simulink subsystem "Average_SEPIC"  (R2021b)
settings: Solver=VariableStepAuto  StartTime=0.0  StopTime=0.5  RelTol=1e-3
undefined symbols (not defined in the file): D1_Rs, D1_Vf, PR1_Res, R9_Res
libraries: fl_lib x23, ee_lib x7, nesl_utility x5, simulink x1
settings Model: DefaultTestHarness=DCDC_SEPIC_Pulse0_61_LED0  Creator=vlenzi  LastModifiedBy=vlenzi
settings SolverCC: AlgebraicLoopSolver=TrustRegion
settings DebuggingCC: SFMachineParentedDataDiag=warning

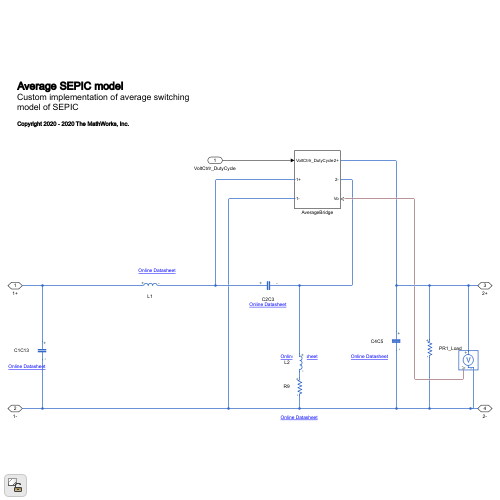
[thumbnail: Simulink's stored preview of the top-level diagram]
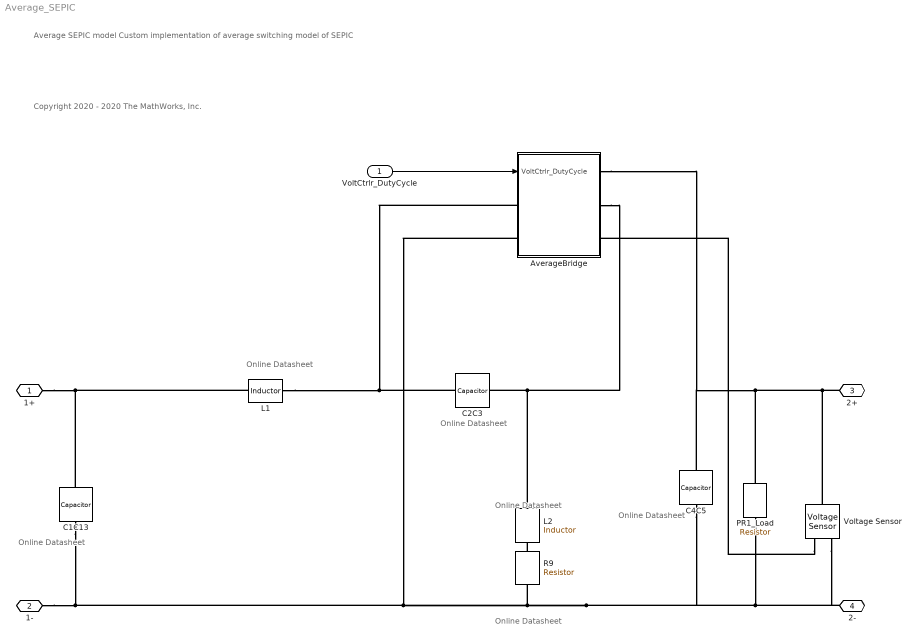
== system Average_SEPIC ==
  note: Online Datasheet
  note: Online Datasheet
  note: Online Datasheet
  note: Online Datasheet
  note: Online Datasheet
  note: Online Datasheet
  note: Average SEPIC model
      | Custom implementation of average switching model of SEPIC
  note: Copyright 2020 - 2020 The MathWorks, Inc.
  VoltCtrlr_DutyCycle : Inport  Unit=1  PortDimensions=1
  AverageBridge : Subsystem
  C1C13 : ee_lib/Passive/Capacitor  cap_option=0  c=C1C13_Cap uF  Cvec=[1e-05, 1e-06] F  Vvec=[0, 10] V  CV_table_symmetry=1  f_vec=[1, 10] kHz  DFext_vec=[.8, 1.2]  C_tol=C1C13_Tol  enable_C_tol=0  tol_distribution=1  nSigma=4  r=1e-6 Ohm  g=0 1/Ohm  averaging_period=0 s  enable_operating_limits=0  operating_limit_action=2  max_working_voltage_range=[-25, 25] V  power_rating=1 W  enable_faults=0  fault_action=1  Cscale_faulted=100  R_faulted=1e-3 Ohm  G_faulted=0 1/Ohm  tau_fault=1e-3 s  enable_temporal_fault=0  t_fault=1 s  enable_behavioral_fault=0  max_permissible_voltage_range=[-100, 100] V  t_fail_on_voltage=1 s  i_specify=off  i_priority=None  i=0 A  i_nominal_specify=off  i_nominal_unit=A  i_nominal_value=1  v_specify=off  v_priority=None  v=0 V  v_nominal_specify=off  v_nominal_unit=V  v_nominal_value=1  vc_specify=off  vc_priority=High  vc=0 V  vc_nominal_specify=off  vc_nominal_unit=V  vc_nominal_value=1
  C2C3 : ee_lib/Passive/Capacitor  cap_option=0  c=C2C3_Cap uF  Cvec=[1e-05, 1e-06] F  Vvec=[0, 10] V  CV_table_symmetry=1  f_vec=[1, 10] kHz  DFext_vec=[.8, 1.2]  C_tol=C2C3_Tol  enable_C_tol=0  tol_distribution=1  nSigma=4  r=1e-6 Ohm  g=0 1/Ohm  averaging_period=0 s  enable_operating_limits=0  operating_limit_action=2  max_working_voltage_range=[-25, 25] V  power_rating=1 W  enable_faults=0  fault_action=1  Cscale_faulted=100  R_faulted=1e-3 Ohm  G_faulted=0 1/Ohm  tau_fault=1e-3 s  enable_temporal_fault=0  t_fault=1 s  enable_behavioral_fault=0  max_permissible_voltage_range=[-100, 100] V  t_fail_on_voltage=1 s  i_specify=off  i_priority=None  i=0 A  i_nominal_specify=off  i_nominal_unit=A  i_nominal_value=1  v_specify=off  v_priority=High  v=psu_V V  v_nominal_specify=off  v_nominal_unit=V  v_nominal_value=1  vc_specify=off  vc_priority=High  vc=0 V  vc_nominal_specify=off  vc_nominal_unit=V  vc_nominal_value=1
  C4C5 : ee_lib/Passive/Capacitor  cap_option=0  c=C4C5_Cap uF  Cvec=[1e-05, 1e-06] F  Vvec=[0, 10] V  CV_table_symmetry=1  f_vec=[1, 10] kHz  DFext_vec=[.8, 1.2]  C_tol=C4C5_Tol  enable_C_tol=0  tol_distribution=1  nSigma=4  r=1e-6 Ohm  g=0 1/Ohm  averaging_period=0 s  enable_operating_limits=0  operating_limit_action=2  max_working_voltage_range=[-25, 25] V  power_rating=1 W  enable_faults=0  fault_action=1  Cscale_faulted=100  R_faulted=1e-3 Ohm  G_faulted=0 1/Ohm  tau_fault=1e-3 s  enable_temporal_fault=0  t_fault=1 s  enable_behavioral_fault=0  max_permissible_voltage_range=[-100, 100] V  t_fail_on_voltage=1 s  i_specify=off  i_priority=None  i=0 A  i_nominal_specify=off  i_nominal_unit=A  i_nominal_value=1  v_specify=off  v_priority=None  v=0 V  v_nominal_specify=off  v_nominal_unit=V  v_nominal_value=1  vc_specify=off  vc_priority=High  vc=0 V  vc_nominal_specify=off  vc_nominal_unit=V  vc_nominal_value=1
  L1 : ee_lib/Passive/Inductor  l=L1_Ind uH  L_tol=L1_Tol  enable_L_tol=0  tol_distribution=1  nSigma=4  r=L1_Res Ohm  g=0 1/Ohm  enable_operating_limits=0  operating_limit_action=2  max_working_current=1 A  power_rating=1 W  enable_faults=0  fault_action=1  lambdaPercent=50  k_faulted=0.9999  turnsShort=0  openCct=0  groundShort=0  groundShortG=0 1/Ohm  tau_fault=1e-3 s  enable_temporal_fault=0  t_fault=1 s  enable_behavioral_fault=0  max_permissible_voltage=100 V  n_fail_on_voltage=1  max_permissible_current=1 A  t_fail_on_current=1 s  i_L_specify=off  i_L_priority=High  i_L=0 A  i_L_nominal_specify=off  i_L_nominal_unit=A  i_L_nominal_value=1
  L2 : ee_lib/Passive/Inductor  l=L2_Ind uH  L_tol=L2_Tol  enable_L_tol=0  tol_distribution=1  nSigma=4  r=L2_Res Ohm  g=0 1/Ohm  enable_operating_limits=0  operating_limit_action=2  max_working_current=1 A  power_rating=1 W  enable_faults=0  fault_action=1  lambdaPercent=50  k_faulted=0.9999  turnsShort=0  openCct=0  groundShort=0  groundShortG=0 1/Ohm  tau_fault=1e-3 s  enable_temporal_fault=0  t_fault=1 s  enable_behavioral_fault=0  max_permissible_voltage=100 V  n_fail_on_voltage=1  max_permissible_current=1 A  t_fail_on_current=1 s  i_L_specify=off  i_L_priority=High  i_L=0 A  i_L_nominal_specify=off  i_L_nominal_unit=A  i_L_nominal_value=1
  PR1_Load : ee_lib/Passive/Resistor  R=PR1_Res Ohm  R_tol=PR1_Tol  enable_R_tol=0  tol_distribution=1  nSigma=4  enable_operating_limits=0  operating_limit_action=2  max_working_voltage=100 V  power_rating=1 W  enable_faults=0  fault_action=1  R_faulted=inf Ohm  enable_temporal_fault=0  t_fault=1 s  enable_behavioral_fault=0  max_permissible_current=1 A  t_fail_on_current=1 s  noise_mode=0  sample_time=1e-3 s  repeatability=1  auto_seed=3118594787  user_seed=0  Tdevice=25 degC  power_derating_T1=70 degC  power_derating_T2=155 degC  operating_temperature_range_vec=[-50, 150] degC  alpha=3.93e-3 1/K  Tmeas=25 degC  thermal_mass=100 J/K  temperature_specify=off  temperature_priority=High  temperature=298.15 K  temperature_nominal_specify=off  temperature_nominal_unit=K  temperature_nominal_value=1
  R9 : ee_lib/Passive/Resistor  R=R9_Res Ohm  R_tol=R9_Tol  enable_R_tol=0  tol_distribution=1  nSigma=4  enable_operating_limits=0  operating_limit_action=2  max_working_voltage=100 V  power_rating=1 W  enable_faults=0  fault_action=1  R_faulted=inf Ohm  enable_temporal_fault=0  t_fault=1 s  enable_behavioral_fault=0  max_permissible_current=1 A  t_fail_on_current=1 s  noise_mode=0  sample_time=1e-3 s  repeatability=1  auto_seed=3362409950  user_seed=0  Tdevice=25 degC  power_derating_T1=70 degC  power_derating_T2=155 degC  operating_temperature_range_vec=[-50, 150] degC  alpha=3.93e-3 1/K  Tmeas=25 degC  thermal_mass=100 J/K  temperature_specify=off  temperature_priority=High  temperature=298.15 K  temperature_nominal_specify=off  temperature_nominal_unit=K  temperature_nominal_value=1
  Voltage Sensor : fl_lib/Electrical/Electrical Sensors/Voltage Sensor
  1+ : PMIOPort  Side=Left
  1- : PMIOPort  Port=2  Side=Left
  2+ : PMIOPort  Port=3  Side=Right
  2- : PMIOPort  Port=4  Side=Right
  wires:
  VoltCtrlr_DutyCycle/1 -> AverageBridge/1(VoltCtrlr_DutyCycle)
  connections:
  Voltage Sensor/LConn1 -- AverageBridge/RConn1 -- C4C5/LConn1 -- PR1_Load/LConn1 -- 2+/RConn1
  L1/LConn1 -- C1C13/LConn1 -- 1+/RConn1
  1-/RConn1 -- 2-/RConn1 -- Voltage Sensor/RConn2 -- PR1_Load/RConn1 -- C4C5/RConn1 -- R9/RConn1 -- AverageBridge/LConn2 -- C1C13/RConn1
  AverageBridge/LConn1 -- C2C3/LConn1 -- L1/RConn1
  L2/LConn1 -- C2C3/RConn1 -- AverageBridge/RConn2
  R9/LConn1 -- L2/RConn1
  Voltage Sensor/RConn1 -- AverageBridge/RConn3

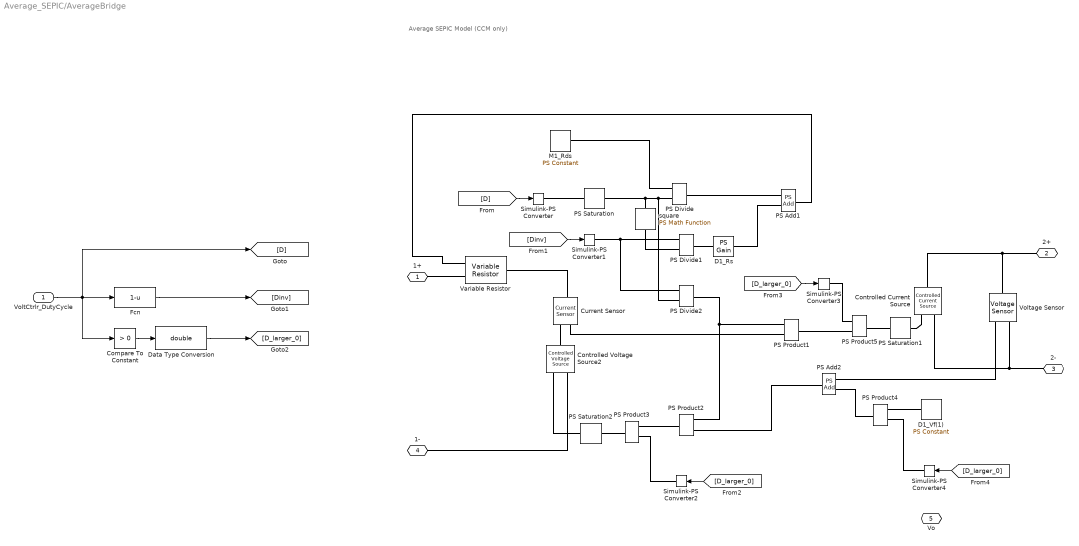
== system Average_SEPIC/AverageBridge ==
  note: Average SEPIC Model (CCM only)
  VoltCtrlr_DutyCycle : Inport  Unit=1  PortDimensions=1
  Compare To Constant : simulink/Logic and Bit Operations/Compare To Constant  relop=>  const=0  OutDataTypeStr=uint8
  Controlled Current Source : fl_lib/Electrical/Electrical Sources/Controlled Current Source
  Controlled Voltage Source2 : fl_lib/Electrical/Electrical Sources/Controlled Voltage Source
  Current Sensor : fl_lib/Electrical/Electrical Sensors/Current Sensor
  D1_Rs : fl_lib/Physical Signals/Functions/PS Gain  gain=D1_Rs Ohm
  D1_Vf(1) : fl_lib/Physical Signals/Sources/PS Constant  constant=D1_Vf(1) V
  Data Type Conversion : DataTypeConversion  OutDataTypeStr=double
  Fcn : Fcn  Expr=1-u
  M1_Rds : fl_lib/Physical Signals/Sources/PS Constant  constant=M1_Rds Ohm
  PS Add1 : fl_lib/Physical Signals/Functions/PS Add
  PS Add2 : fl_lib/Physical Signals/Functions/PS Add
  PS Divide : fl_lib/Physical Signals/Functions/PS Divide
      settings: SourceProductBaseCode=SS
  PS Divide1 : fl_lib/Physical Signals/Functions/PS Divide
      settings: SourceProductBaseCode=SS
  PS Divide2 : fl_lib/Physical Signals/Functions/PS Divide
      settings: SourceProductBaseCode=SS
  PS Product{1..5} (5 alike) : fl_lib/Physical Signals/Functions/PS Product
  PS Saturation : fl_lib/Physical Signals/Nonlinear Operators/PS Saturation  upper_limit=inf  lower_limit=1e-5
      settings: SourceProductBaseCode=SS
  PS Saturation1 : fl_lib/Physical Signals/Nonlinear Operators/PS Saturation  upper_limit=inf A  lower_limit=0 A
      settings: SourceProductBaseCode=SS
  PS Saturation2 : fl_lib/Physical Signals/Nonlinear Operators/PS Saturation  upper_limit=inf V  lower_limit=0 V
      settings: SourceProductBaseCode=SS
  Simulink-PS Converter{,1..4} (5 alike) : nesl_utility/Simulink-PS Converter  PhysicalDomain=network_engine_domain  SubClassName=ps_input  LeftPortType=input  RightPortType=output  PseudoPeriodic=off  Frequencies=[]  NoiseDistribution=none  NoiseParameters=[]  Unit=1  AffineConversion=off  FilteringAndDerivatives=provide  SimscapeFilterOrder=1  InputFilterTimeConstant=0.001  UdotUserProvided=0
      settings: SourceProductBaseCode=PW,SS
  Variable Resistor : fl_lib/Electrical/Electrical Elements/Variable Resistor  Rmin=0 Ohm  i_specify=off  i_priority=None  i=0 A  i_nominal_specify=off  i_nominal_unit=A  i_nominal_value=1  v_specify=off  v_priority=None  v=0 V  v_nominal_specify=off  v_nominal_unit=V  v_nominal_value=1
  Voltage Sensor : fl_lib/Electrical/Electrical Sensors/Voltage Sensor
  square : fl_lib/Physical Signals/Functions/PS Math Function  fcn_choice=foundation.enum.math_function.square  v=1
      settings: SourceProductBaseCode=SS
  1+ : PMIOPort  Side=Left
  2+ : PMIOPort  Port=2  Side=Right
  2- : PMIOPort  Port=3  Side=Right
  1- : PMIOPort  Port=4  Side=Left
  Vo : PMIOPort  Port=5  Side=Right
  wires:
  VoltCtrlr_DutyCycle/1 -> Compare To Constant/1, Fcn/1, [D]
  Fcn/1 -> [Dinv]
  Compare To Constant/1 -> Data Type Conversion/1
  Data Type Conversion/1 -> [D_larger_0]
  [D] -> Simulink-PS Converter/1
  [Dinv] -> Simulink-PS Converter1/1
  [D_larger_0] -> Simulink-PS Converter2/1
  [D_larger_0] -> Simulink-PS Converter3/1
  [D_larger_0] -> Simulink-PS Converter4/1
  connections:
  Current Sensor/RConn1 -- PS Product1/LConn2
  PS Add2/RConn1 -- PS Product2/LConn1
  PS Divide2/RConn1 -- PS Product1/LConn1 -- PS Product2/LConn2
  Variable Resistor/LConn1 -- PS Add1/RConn1
  Variable Resistor/RConn1 -- Current Sensor/LConn1
  1+/RConn1 -- Variable Resistor/LConn2
  D1_Rs/RConn1 -- PS Add1/LConn2
  PS Divide1/LConn2 -- square/RConn1
  PS Divide1/RConn1 -- D1_Rs/LConn1
  PS Add1/LConn1 -- PS Divide/RConn1
  M1_Rds/RConn1 -- PS Divide/LConn1
  PS Product3/RConn1 -- PS Saturation2/LConn1
  PS Add2/LConn2 -- Voltage Sensor/RConn1
  Voltage Sensor/RConn2 -- Controlled Current Source/RConn2 -- 2-/RConn1
  Voltage Sensor/LConn1 -- Controlled Current Source/LConn1 -- 2+/RConn1
  PS Divide2/LConn2 -- PS Divide/LConn2 -- PS Saturation/RConn1 -- square/LConn1
  PS Saturation/LConn1 -- Simulink-PS Converter/RConn1
  Controlled Voltage Source2/RConn2 -- 1-/RConn1
  Controlled Current Source/RConn1 -- PS Saturation1/RConn1
  Current Sensor/RConn2 -- Controlled Voltage Source2/LConn1
  PS Divide2/LConn1 -- PS Divide1/LConn1 -- Simulink-PS Converter1/RConn1
  PS Saturation2/RConn1 -- Controlled Voltage Source2/RConn1
  PS Product3/LConn2 -- PS Product2/RConn1
  Simulink-PS Converter2/RConn1 -- PS Product3/LConn1
  PS Product4/RConn1 -- PS Add2/LConn1
  PS Product5/RConn1 -- PS Saturation1/LConn1
  PS Product1/RConn1 -- PS Product5/LConn2
  Simulink-PS Converter3/RConn1 -- PS Product5/LConn1
  D1_Vf(1)/RConn1 -- PS Product4/LConn2
  Simulink-PS Converter4/RConn1 -- PS Product4/LConn1
